simulink model "MECROKA_TWR_B"  (R2017b)
settings: Solver=FixedStepDiscrete  StartTime=0.0  StopTime=inf  RelTol=1e-3  EnableMultiTasking=on
InitFcn:
  | % BLDC-data
  | num_pol_pairs = 7
  | res_period = 5000;
  | res_pwm   = 2^8;
  | 
  | wheel_radius=0.033;
  | axle_length=0.2;
undefined symbols (not defined in the file): DiscIntNeverNeededParam
libraries: MecRoKa_SFunction_Library x18, arduinolib x12, simulink x5, simulink_extras x2
(part 2 of 2)

== stateflow chart MECROKA_TWR_B/autonomous targets ==
  state stop11 [commented out]
    en: pos_vel_flag = 0;
    en, du: vel_trgt_auto   = 0.0;
    en, du: yaw_rate_trgt_auto  = 0.0;
    en, du: pos_trgt_auto = 0.0;
  state reset [commented out]
    en: pos_vel_flag = 0;
  state go_forward [commented out]
    en, du: vel_trgt_auto   = 0.0;
    en, du: yaw_rate_trgt_auto  = 0.0;
    en, du: pos_trgt_auto = 3;
    en, du: pos_vel_flag = 1;
  state set_autonomous_targets
    state Operation_mode_1
      en, du: pos_vel_flag = 0;
      state stop1
        en, du: vel_trgt_auto   = 0.0;
        en, du: yaw_rate_trgt_auto  = 0.0;
        en, du: pos_trgt_auto = 0.0;
      state go_forward_acc
        en, du: vel_trgt_auto   = 0.6;
        en, du: yaw_rate_trgt_auto  = 0.0;
        en, du: pos_trgt_auto = 0;
      state go_backward_acc
        en, du: vel_trgt_auto   = 0.4;
        en, du: yaw_rate_trgt_auto  = 0.0;
        en, du: pos_trgt_auto = 0;
      state stop2
        en, du: vel_trgt_auto   = 0.0;
        en, du: yaw_rate_trgt_auto  = 0.0;
        en: pos_trgt_auto = 1;
      state reset1
        en: pos_vel_flag = 1;
      (default) -> set_autonomous_targets.Operation_mode_1.stop1
      set_autonomous_targets.Operation_mode_1.stop1 -> go_forward_acc : after(3,sec)
      go_forward_acc -> go_backward_acc : after(8,sec)
      go_backward_acc -> set_autonomous_targets.Operation_mode_1.stop2 : after(1,sec)
      set_autonomous_targets.Operation_mode_1.stop2 -> set_autonomous_targets.Operation_mode_1.reset1 : after(0.25,sec)
      set_autonomous_targets.Operation_mode_1.reset1 -> Operation_mode_1 : after(100,sec)
    state Operation_mode_2
      state stop1
        en: pos_vel_flag = 0;
        en, du: vel_trgt_auto   = 0.00;
        en, du: yaw_rate_trgt_auto  = 0.0;
      state reset1
        en: pos_vel_flag = 0;
      state go_forward1
        en, du: vel_trgt_auto   = 0.0;
        en, du: yaw_rate_trgt_auto  =0;
        en, du: pos_trgt_auto = 0.75;
        en, du: pos_vel_flag = 1;
      state stop2
        en: pos_vel_flag = 0;
        en, du: vel_trgt_auto   = 0.00;
        en, du: yaw_rate_trgt_auto  = 0.0;
      state reset2
        en: pos_vel_flag = 0;
      state go_rotate1
        en, du: vel_trgt_auto   = 0.0;
        en, du: yaw_rate_trgt_auto  = 0.985*pi;
        en, du: pos_vel_flag = 0;
      state go_rotate2
        en, du: vel_trgt_auto   = 0.0;
        en, du: yaw_rate_trgt_auto  = 0.985*pi;
        en, du: pos_vel_flag = 0;
      state stop3
        en, du: vel_trgt_auto   = 0.00;
        en, du: yaw_rate_trgt_auto  = 0.0;
        en, du: pos_vel_flag = 0;
      state reset3
        en: pos_vel_flag = 0;
      state go_forward2
        en, du: vel_trgt_auto   = 0.0;
        en, du: yaw_rate_trgt_auto  =0;
        en, du: pos_trgt_auto = 0.75;
        en, du: pos_vel_flag = 1;
      state stop4
        en: pos_vel_flag = 0;
        en, du: vel_trgt_auto   = 0.00;
        en, du: yaw_rate_trgt_auto  = 0.0;
      state reset4
        en: pos_vel_flag = 0;
      state go_rotate3
        en, du: vel_trgt_auto   = 0.0;
        en, du: yaw_rate_trgt_auto  = 0.986*pi;
        en, du: pos_vel_flag = 0;
      state go_rotate4
        en, du: vel_trgt_auto   = 0.0;
        en, du: yaw_rate_trgt_auto  = 0.986*pi;
        en, du: pos_vel_flag = 0;
      state stop5
        en, du: vel_trgt_auto   = 0.00;
        en, du: yaw_rate_trgt_auto  = 0.0;
        en, du: pos_vel_flag = 0;
      state reset5
        en: pos_vel_flag = 0;
      state go_forward3
        en, du: vel_trgt_auto   = 0.0;
        en, du: yaw_rate_trgt_auto  =0;
        en, du: pos_trgt_auto = 0.75;
        en, du: pos_vel_flag = 1;
      state stop6
        en: pos_vel_flag = 0;
        en, du: vel_trgt_auto   = 0.00;
        en, du: yaw_rate_trgt_auto  = 0.0;
      state reset6
        en: pos_vel_flag = 0;
      state go_rotate5
        en, du: vel_trgt_auto   = 0.0;
        en, du: yaw_rate_trgt_auto  = 0.987*pi;
        en, du: pos_vel_flag = 0;
      state go_rotate6
        en, du: vel_trgt_auto   = 0.0;
        en, du: yaw_rate_trgt_auto  = 0.987*pi;
        en, du: pos_vel_flag = 0;
      state stop7
        en, du: vel_trgt_auto   = 0.00;
        en, du: yaw_rate_trgt_auto  = 0.0;
        en, du: pos_vel_flag = 0;
      state reset7
        en: pos_vel_flag = 0;
      state go_forward4
        en, du: vel_trgt_auto   = 0.0;
        en, du: yaw_rate_trgt_auto  =0;
        en, du: pos_trgt_auto = 0.75;
        en, du: pos_vel_flag = 1;
      state stop8
        en: pos_vel_flag = 0;
        en, du: vel_trgt_auto   = 0.00;
        en, du: yaw_rate_trgt_auto  = 0.0;
      state reset8
        en: pos_vel_flag = 0;
      (default) -> set_autonomous_targets.Operation_mode_2.stop1
      set_autonomous_targets.Operation_mode_2.stop1 -> set_autonomous_targets.Operation_mode_2.reset1 : after(5,sec)
      set_autonomous_targets.Operation_mode_2.reset1 -> go_forward1
      go_forward1 -> set_autonomous_targets.Operation_mode_2.stop2 : after(2.5,sec)
      set_autonomous_targets.Operation_mode_2.stop2 -> set_autonomous_targets.Operation_mode_2.reset2 : after(1,sec)
      set_autonomous_targets.Operation_mode_2.reset2 -> go_rotate1
      go_rotate1 -> set_autonomous_targets.Operation_mode_2.go_rotate2 : after(1,sec)
      set_autonomous_targets.Operation_mode_2.go_rotate2 -> set_autonomous_targets.Operation_mode_2.stop3 : after(1,sec)
      set_autonomous_targets.Operation_mode_2.stop3 -> set_autonomous_targets.Operation_mode_2.reset3 : after(1,sec)
      set_autonomous_targets.Operation_mode_2.reset3 -> set_autonomous_targets.Operation_mode_2.go_forward2
      set_autonomous_targets.Operation_mode_2.go_forward2 -> set_autonomous_targets.Operation_mode_2.stop4 : after(2.3,sec)
      set_autonomous_targets.Operation_mode_2.stop4 -> reset4 : after(1,sec)
      reset4 -> set_autonomous_targets.Operation_mode_2.go_rotate3
      set_autonomous_targets.Operation_mode_2.go_rotate3 -> go_rotate4 : after(1,sec)
      go_rotate4 -> set_autonomous_targets.Operation_mode_2.stop5 : after(1,sec)
      set_autonomous_targets.Operation_mode_2.stop5 -> reset5 : after(1,sec)
      reset5 -> set_autonomous_targets.Operation_mode_2.go_forward3
      set_autonomous_targets.Operation_mode_2.go_forward3 -> set_autonomous_targets.Operation_mode_2.stop6 : after(2.2,sec)
      set_autonomous_targets.Operation_mode_2.stop6 -> reset6 : after(1,sec)
      reset6 -> set_autonomous_targets.Operation_mode_2.go_rotate5
      set_autonomous_targets.Operation_mode_2.go_rotate5 -> set_autonomous_targets.Operation_mode_2.go_rotate6 : after(1,sec)
      set_autonomous_targets.Operation_mode_2.go_rotate6 -> set_autonomous_targets.Operation_mode_2.stop7 : after(1,sec)
      set_autonomous_targets.Operation_mode_2.stop7 -> reset7 : after(1,sec)
      reset7 -> set_autonomous_targets.Operation_mode_2.go_forward4
      set_autonomous_targets.Operation_mode_2.go_forward4 -> set_autonomous_targets.Operation_mode_2.stop8 : after(2.5,sec)
      set_autonomous_targets.Operation_mode_2.stop8 -> reset8
      reset8 -> Operation_mode_2 : after(100,sec)
    state Operation_mode_3
      state stop1
        en: pos_vel_flag = 0;
        en, du: vel_trgt_auto   = 0.0;
        en, du: yaw_rate_trgt_auto  = 0.0;
        en, du: pos_trgt_auto = 0.0;
      state reset
        en: pos_vel_flag = 0;
      state go_forward
        en, du: vel_trgt_auto   = 0.0;
        en, du: yaw_rate_trgt_auto  = 0.0;
        en, du: pos_trgt_auto = 0;
        en, du: pos_vel_flag = 1;
      (default) -> set_autonomous_targets.Operation_mode_3.stop1
      set_autonomous_targets.Operation_mode_3.stop1 -> set_autonomous_targets.Operation_mode_3.reset : after(3,sec)
      set_autonomous_targets.Operation_mode_3.reset -> set_autonomous_targets.Operation_mode_3.go_forward
      set_autonomous_targets.Operation_mode_3.go_forward -> Operation_mode_3 : after(150,sec)
    state Operation_mode_4
      en, du: pos_vel_flag = 0;
      state stop1
        en: pos_vel_flag = 0;
        en, du: vel_trgt_auto   = 0.0;
        en, du: yaw_rate_trgt_auto  = 0.0;
      state stop2
        en: pos_vel_flag = 0;
        en, du: vel_trgt_auto   = 0.62;
        en, du: yaw_rate_trgt_auto  = pi/4;
      state stop3
        en: pos_vel_flag = 0;
        en, du: vel_trgt_auto   = 0.62;
        en, du: yaw_rate_trgt_auto  = -pi/4;
      state stop4
        en: pos_vel_flag = 0;
        en, du: vel_trgt_auto   = 0.0;
        en, du: yaw_rate_trgt_auto  = 0.0;
      (default) -> set_autonomous_targets.Operation_mode_4.stop1
      set_autonomous_targets.Operation_mode_4.stop1 -> set_autonomous_targets.Operation_mode_4.stop2 : after(3,sec)
      set_autonomous_targets.Operation_mode_4.stop2 -> set_autonomous_targets.Operation_mode_4.stop3 : after(7.8,sec)
      set_autonomous_targets.Operation_mode_4.stop3 -> set_autonomous_targets.Operation_mode_4.stop4 : after(7.8,sec)
      set_autonomous_targets.Operation_mode_4.stop4 -> Operation_mode_4 : after(100,sec)
    state OP_mode_off_0
      en, du: vel_trgt_auto   = 0.00;
      en, du: yaw_rate_trgt_auto  = 0.0;
      en, du: pos_trgt_auto = 0;
      en, du: pos_vel_flag = 1;
    Operation_mode_1 -> set_autonomous_targets : [op_mode ~= 1]
    (default) -> (junction 59)
    (junction 59) -> Operation_mode_1 [order 1] : [op_mode == 1]
    (junction 59) -> (junction 156) [order 2]
    (junction 156) -> (junction 61)
    (junction 61) -> Operation_mode_3 [order 1] : [op_mode == 3]
    (junction 61) -> (junction 224) [order 2]
    Operation_mode_3 -> set_autonomous_targets : [op_mode ~= 3]
    Operation_mode_2 -> set_autonomous_targets : [op_mode ~= 2]
    (junction 224) -> Operation_mode_2 [order 1] : [op_mode == 2]
    (junction 224) -> (junction 305) [order 2]
    (junction 305) -> Operation_mode_4 [order 1] : [op_mode == 4]
    Operation_mode_4 -> set_autonomous_targets : [op_mode ~= 4]
    (junction 305) -> (junction 151) [order 2]
    (junction 151) -> OP_mode_off_0
    OP_mode_off_0 -> set_autonomous_targets
  state stop12 [commented out]
    en, du: vel_trgt_auto   = 0.0;
    en, du: yaw_rate_trgt_auto  = 0.0;
    en, du: pos_trgt_auto = 0;
    en, du: pos_vel_flag = 0;
  state go_forward2 [commented out]
    en, du: vel_trgt_auto   = 0.6;
    en, du: yaw_rate_trgt_auto  =0;
  state stop10 [commented out]
    en, du: vel_trgt_auto   = 0.0;
    en, du: yaw_rate_trgt_auto  = 0.0;
    en, du: pos_trgt_auto = 0;
    en, du: pos_vel_flag = 0;
  state stop5 [commented out]
    en, du: vel_trgt_auto   = 0.00;
    en, du: yaw_rate_trgt_auto  = 0.0;
  state go_rotate2 [commented out]
    en, du: vel_trgt_auto   = 0.0;
    en, du: yaw_rate_trgt_auto  = 0.985*pi;
  state go_rotate5 [commented out]
    en, du: vel_trgt_auto   = 0.0;
    en, du: yaw_rate_trgt_auto  = 0.985*pi;
  state reset2 [commented out]
    en: pos_vel_flag = 1;
  state stop8 [commented out]
    en, du: vel_trgt_auto   = 0.00;
    en, du: yaw_rate_trgt_auto  = 0.0;
  state stop9 [commented out]
    en, du: vel_trgt_auto   = 0.0;
    en, du: yaw_rate_trgt_auto  = 0.0;
    en, du: pos_trgt_auto = 0;
    en, du: pos_vel_flag = 1;
  state go_forward3 [commented out]
    en, du: vel_trgt_auto   = 0.6;
    en, du: yaw_rate_trgt_auto  =0;
  state stop6 [commented out]
    en, du: vel_trgt_auto   = 0.00;
    en, du: yaw_rate_trgt_auto  = 0.0;
  state go_rotate3 [commented out]
    en, du: vel_trgt_auto   = 0.0;
    en, du: yaw_rate_trgt_auto  = 0.985*pi;
  state go_rotate6 [commented out]
    en, du: vel_trgt_auto   = 0.0;
    en, du: yaw_rate_trgt_auto  = 0.985*pi;
  state stop7 [commented out]
    en, du: vel_trgt_auto   = 0.00;
    en, du: yaw_rate_trgt_auto  = 0.0;
  state reset3 [commented out]
    en, du: pos_vel_flag = 0;
  state go_forward4 [commented out]
    en, du: vel_trgt_auto   = 0.7;
    en, du: yaw_rate_trgt_auto  =0;
  state stop3 [commented out]
    en, du: vel_trgt_auto   = 0.00;
    en, du: yaw_rate_trgt_auto  = 0.0;
  (default) -> stop11 [commented out]
  stop11 -> reset [commented out] : after(3,sec)
  reset -> go_forward [commented out]
  (default) -> set_autonomous_targets
  go_forward -> stop12 [commented out] : after(150,sec)
  stop12 -> ? [commented out]
  (default) -> go_forward2 [commented out] : after(1,sec)
  go_forward2 -> stop5 [commented out] : after(5,sec)
  stop5 -> go_rotate2 [commented out] : after(1,sec)
  go_rotate2 -> go_rotate5 [commented out] : after(1,sec)
  (default) -> reset2 [commented out]
  go_rotate5 -> stop8 [commented out] : after(1,sec)
  reset2 -> stop9 [commented out]
  stop8 -> go_forward3 [commented out] : after(1,sec)
  go_forward3 -> stop6 [commented out] : after(5,sec)
  stop6 -> go_rotate3 [commented out] : after(1,sec)
  go_rotate3 -> go_rotate6 [commented out] : after(1,sec)
  go_rotate6 -> stop7 [commented out] : after(1,sec)
  (default) -> reset3 [commented out]
  stop7 -> go_forward4 [commented out] : after(1,sec)
  go_forward4 -> stop3 [commented out] : after(4,sec)
  reset3 -> ? [commented out] : after(100,sec)
  data: op_mode input uint8 size=1; vel_trgt_auto output double size=1; yaw_rate_trgt_auto output double size=1; pos_trgt_auto output double size=1; pos_vel_flag output double size=1
  events: t_fc_auto_trgts input FUNCTION_CALL_EVENT

== stateflow chart MECROKA_TWR_B/Mavlink Communication ==
  state mavlink_out
    (history)
    state nothing
    state write_heartbeat
      en: write_mavlink_heartbeat();
    state write_mavlink_heartbeat [function]
    state write_imu
      en:write_mavlink_imu(IMU6000_values);
    state write_mavlink_imu(imu_values) [function]
    state write_attitude
      en: write_mavlink_attitude(pitch_pitchrate_est);
    state write_mavlink_attitude(pitch_pitchrate_estimated) [function]
    state write_mavlink_servo_raw(pwm_motor,rc_raw) [function] [commented out]
    state write_servo [commented out]
      en: write_mavlink_servo_raw(pwm_to_motor,rc_raw_values);
    (default) -> (junction 14)
    nothing -> (junction 14)
    (junction 14) -> nothing [order 2]
    write_attitude -> (junction 14)
    (junction 14) -> write_heartbeat [order 1] : [flag_mavlink_on == true]
    write_heartbeat -> write_imu
    write_imu -> write_attitude
    write_attitude -> write_servo [commented out]
  data: imu_values function_input int32 size=6; pitch_pitchrate_estimated function_input double size=2; pwm_motor function_input double size=1; rc_raw function_input double size=1; flag_mavlink_on input boolean size=1; IMU6000_values input int32 size=6; pitch_pitchrate_est input
  events: t_fc_mavlink_com input FUNCTION_CALL_EVENT
